simulink subsystem "cmds2forces_map"  (R2024b)
settings: Solver=VariableStepAuto  StartTime=0.0  StopTime=10.0  RelTol=1e-3
undefined symbols (not defined in the file): Parameters
libraries: eeGeneralControl x32, matrix_library x1
settings Model: Creator=thesa  LastModifiedBy=thesa
settings RTWCC: GPUComputeCapability=3.5

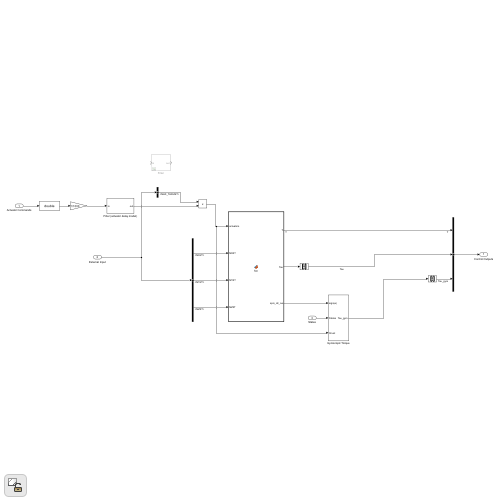
[thumbnail: Simulink's stored preview of the top-level diagram]
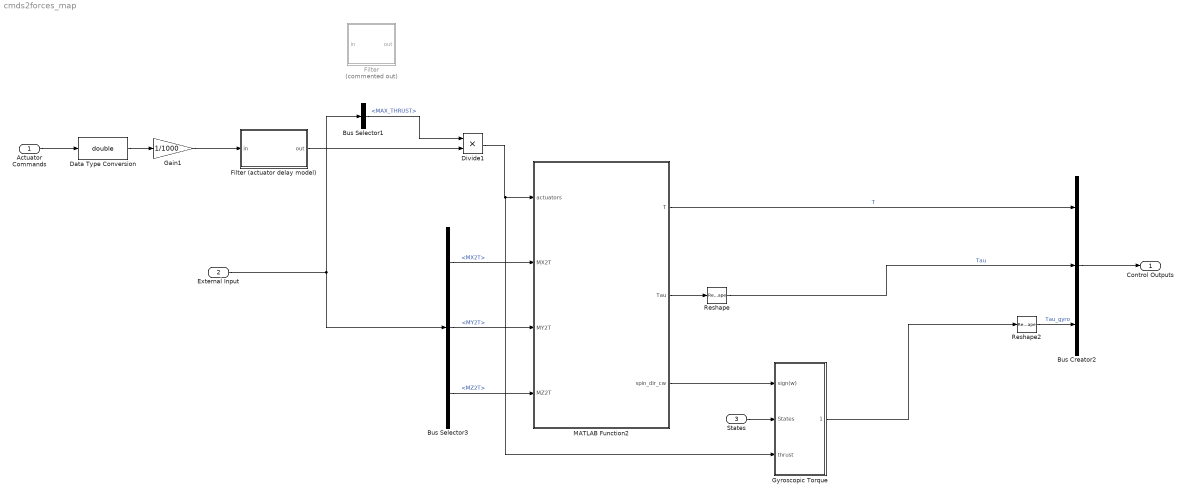
== system cmds2forces_map ==
  Actuator Commands : Inport
  External Input : Inport  Port=2
  States : Inport  Port=3
  Bus Creator2 : BusCreator  Inputs=3
  Bus Selector1 : BusSelector  OutputSignals=Vehicle Parameters.MAX_THRUST
  Bus Selector3 : BusSelector  OutputSignals=Vehicle Parameters.MX2T,Vehicle Parameters.MY2T,Vehicle Parameters.MZ2T
  Data Type Conversion : DataTypeConversion  OutDataTypeStr=double  RndMeth=Convergent  SaturateOnIntegerOverflow=off
  Divide1 : Product  Inputs=**
  Filter : Subsystem  Commented=on
  Filter (actuator delay model) : Subsystem
  Gain1 : Gain  Gain=1/1000
  Gyroscopic Torque : Subsystem
  MATLAB Function2 : MATLAB Function  TreatAsAtomicUnit=on
  Reshape : Reshape  OutputDimensionality=Column vector (2-D)
  Reshape2 : Reshape  OutputDimensionality=Column vector (2-D)
  Control Outputs : Outport
  wires:
  Data Type Conversion/1 -> Gain1/1
  Reshape/1 -> Bus Creator2/2  "Tau"
  MATLAB Function2/1(T) -> Bus Creator2/1  "T"
  External Input/1 -> Bus Selector1/1, Bus Selector3/1
  Filter (actuator delay model)/1(out) -> Divide1/2
  Bus Creator2/1 -> Control Outputs/1
  Actuator Commands/1 -> Data Type Conversion/1
  Bus Selector3/3 -> MATLAB Function2/4(MZ2T)  "<MZ2T>"
  MATLAB Function2/2(Tau) -> Reshape/1
  Divide1/1 -> MATLAB Function2/1(actuators), Gyroscopic Torque/3(thrust)
  Gain1/1 -> Filter (actuator delay model)/1(in)
  Bus Selector3/2 -> MATLAB Function2/3(MY2T)  "<MY2T>"
  Bus Selector1/1 -> Divide1/1  "<MAX_THRUST>"
  Bus Selector3/1 -> MATLAB Function2/2(MX2T)  "<MX2T>"
  Reshape2/1 -> Bus Creator2/3  "Tau_gyro"
  MATLAB Function2/3(spin_dir_cw) -> Gyroscopic Torque/1(sign(w))
  States/1 -> Gyroscopic Torque/2(States)
  Gyroscopic Torque/1(Tau_gyro) -> Reshape2/1

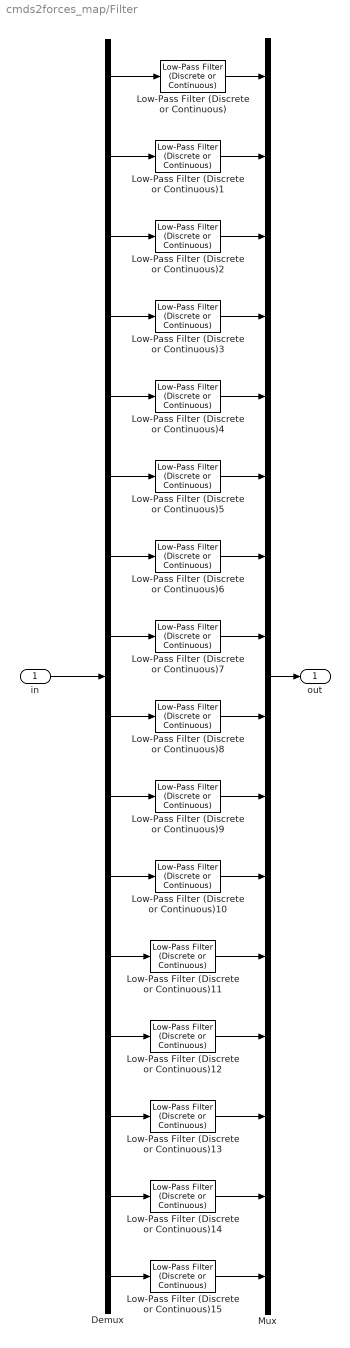
== system cmds2forces_map/Filter ==
  in : Inport
  Demux : Demux  Outputs=16
  Low-Pass Filter (Discrete or Continuous){,1..15} (16 alike) : eeGeneralControl/Low-Pass Filter (Discrete or Continuous)  K=1  T=Parameters.Vehicle.motor_time_constant_s  B=inf  A=-inf  init_option=Inherited from block input  x0=0  Ts=-1
  Mux : Mux  Inputs=16
  out : Outport
  wires:
  Low-Pass Filter (Discrete or Continuous)2/1 -> Mux/3
  Low-Pass Filter (Discrete or Continuous)/1 -> Mux/1
  Demux/3 -> Low-Pass Filter (Discrete or Continuous)2/1
  in/1 -> Demux/1
  Mux/1 -> out/1
  Low-Pass Filter (Discrete or Continuous)1/1 -> Mux/2
  Demux/1 -> Low-Pass Filter (Discrete or Continuous)/1
  Demux/2 -> Low-Pass Filter (Discrete or Continuous)1/1
  Demux/4 -> Low-Pass Filter (Discrete or Continuous)3/1
  Low-Pass Filter (Discrete or Continuous)3/1 -> Mux/4
  Demux/5 -> Low-Pass Filter (Discrete or Continuous)4/1
  Low-Pass Filter (Discrete or Continuous)4/1 -> Mux/5
  Demux/6 -> Low-Pass Filter (Discrete or Continuous)5/1
  Low-Pass Filter (Discrete or Continuous)5/1 -> Mux/6
  Low-Pass Filter (Discrete or Continuous)6/1 -> Mux/7
  Demux/7 -> Low-Pass Filter (Discrete or Continuous)6/1
  Demux/8 -> Low-Pass Filter (Discrete or Continuous)7/1
  Low-Pass Filter (Discrete or Continuous)7/1 -> Mux/8
  Demux/9 -> Low-Pass Filter (Discrete or Continuous)8/1
  Low-Pass Filter (Discrete or Continuous)8/1 -> Mux/9
  Demux/10 -> Low-Pass Filter (Discrete or Continuous)9/1
  Low-Pass Filter (Discrete or Continuous)9/1 -> Mux/10
  Demux/11 -> Low-Pass Filter (Discrete or Continuous)10/1
  Low-Pass Filter (Discrete or Continuous)10/1 -> Mux/11
  Demux/12 -> Low-Pass Filter (Discrete or Continuous)11/1
  Low-Pass Filter (Discrete or Continuous)11/1 -> Mux/12
  Demux/13 -> Low-Pass Filter (Discrete or Continuous)12/1
  Low-Pass Filter (Discrete or Continuous)12/1 -> Mux/13
  Demux/14 -> Low-Pass Filter (Discrete or Continuous)13/1
  Low-Pass Filter (Discrete or Continuous)13/1 -> Mux/14
  Demux/15 -> Low-Pass Filter (Discrete or Continuous)14/1
  Low-Pass Filter (Discrete or Continuous)14/1 -> Mux/15
  Demux/16 -> Low-Pass Filter (Discrete or Continuous)15/1
  Low-Pass Filter (Discrete or Continuous)15/1 -> Mux/16

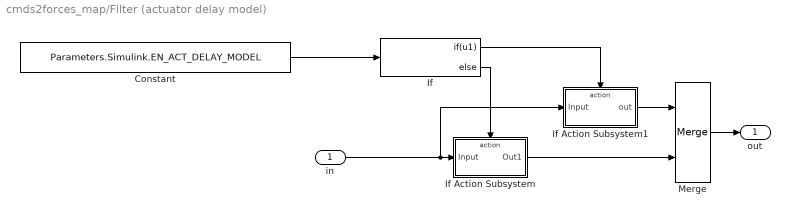
== system cmds2forces_map/Filter (actuator delay model) ==
  in : Inport
  Constant : Constant  Value=Parameters.Simulink.EN_ACT_DELAY_MODEL
  If : If  IfExpression=u1
  If Action Subsystem : Subsystem  TreatAsAtomicUnit=on
  If Action Subsystem1 : Subsystem  TreatAsAtomicUnit=on
  Merge : Merge
  out : Outport
  wires:
  If Action Subsystem/1(Out1) -> Merge/2
  in/1 -> If Action Subsystem/1(Input), If Action Subsystem1/1(Input)
  If Action Subsystem1/1(out) -> Merge/1
  If/2 -> If Action Subsystem/Action
  Constant/1 -> If/1
  If/1 -> If Action Subsystem1/Action
  Merge/1 -> out/1

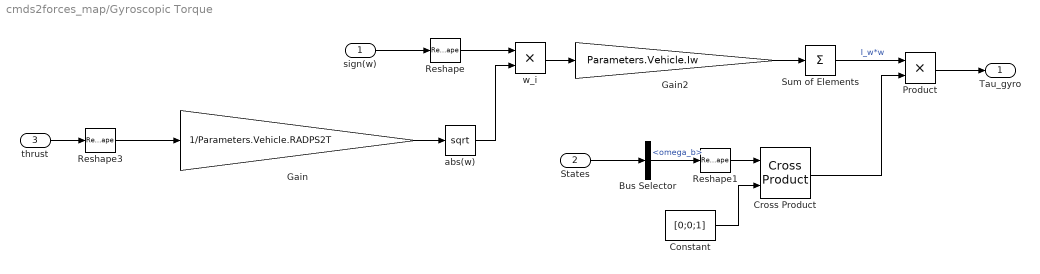
== system cmds2forces_map/Gyroscopic Torque ==
  sign(w) : Inport
  States : Inport  Port=2
  thrust : Inport  Port=3
  Bus Selector : BusSelector  OutputSignals=omega_b
  Constant : Constant  Value=[0;0;1]
  Cross Product : matrix_library/Cross Product
  Gain : Gain  Gain=1/Parameters.Vehicle.RADPS2T
  Gain2 : Gain  Gain=Parameters.Vehicle.Iw
  Product : Product
  Reshape : Reshape
  Reshape1 : Reshape  OutputDimensionality=Column vector (2-D)
  Reshape3 : Reshape
  Sum of Elements : Sum  Inputs=+
  abs(w) : Sqrt  OutputSignalType=real
  w_i : Product  Inputs=**
  Tau_gyro : Outport
  wires:
  sign(w)/1 -> Reshape/1
  Reshape3/1 -> Gain/1
  Gain2/1 -> Sum of Elements/1
  Gain/1 -> abs(w)/1
  Sum of Elements/1 -> Product/1  "I_w*w"
  Cross Product/1 -> Product/2
  Product/1 -> Tau_gyro/1
  w_i/1 -> Gain2/1
  Constant/1 -> Cross Product/2
  abs(w)/1 -> w_i/2
  Reshape/1 -> w_i/1
  Bus Selector/1 -> Reshape1/1  "<omega_b>"
  thrust/1 -> Reshape3/1
  Reshape1/1 -> Cross Product/1
  States/1 -> Bus Selector/1

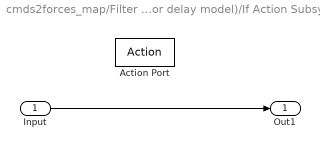
== system cmds2forces_map/Filter (actuator delay model)/If Action Subsystem ==
  Input : Inport
  Action Port : ActionPort  InitializeStates=reset
  Out1 : Outport
  wires:
  Input/1 -> Out1/1

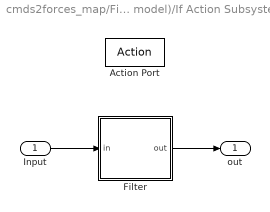
== system cmds2forces_map/Filter (actuator delay model)/If Action Subsystem1 ==
  Input : Inport
  Action Port : ActionPort  InitializeStates=reset
  Filter : Subsystem
  out : Outport
  wires:
  Filter/1(out) -> out/1
  Input/1 -> Filter/1(in)

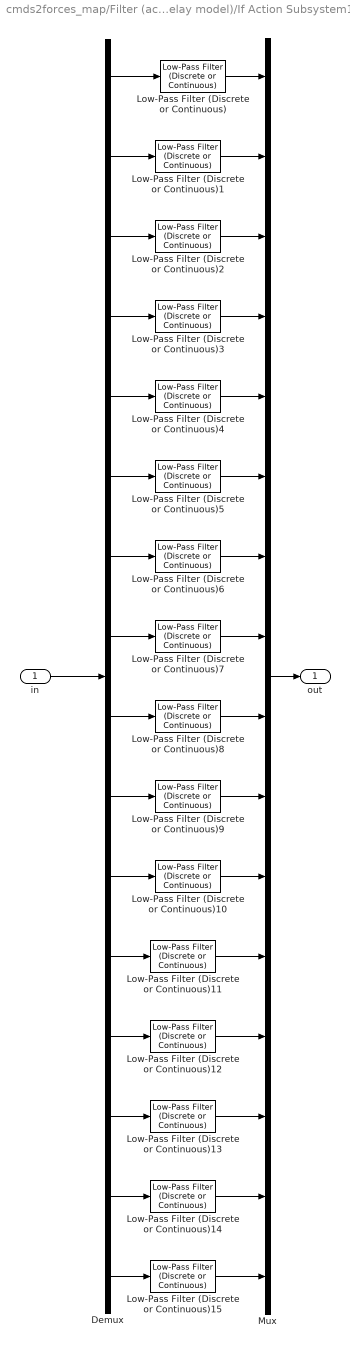
== system cmds2forces_map/Filter (actuator delay model)/If Action Subsystem1/Filter ==
  in : Inport
  Demux : Demux  Outputs=16
  Low-Pass Filter (Discrete or Continuous){,1..15} (16 alike) : eeGeneralControl/Low-Pass Filter (Discrete or Continuous)  K=1  T=Parameters.Vehicle.motor_time_constant_s  B=inf  A=-inf  init_option=Inherited from block input  x0=0  Ts=-1
  Mux : Mux  Inputs=16
  out : Outport
  wires:
  Low-Pass Filter (Discrete or Continuous)2/1 -> Mux/3
  Low-Pass Filter (Discrete or Continuous)/1 -> Mux/1
  Demux/3 -> Low-Pass Filter (Discrete or Continuous)2/1
  in/1 -> Demux/1
  Mux/1 -> out/1
  Low-Pass Filter (Discrete or Continuous)1/1 -> Mux/2
  Demux/1 -> Low-Pass Filter (Discrete or Continuous)/1
  Demux/2 -> Low-Pass Filter (Discrete or Continuous)1/1
  Demux/4 -> Low-Pass Filter (Discrete or Continuous)3/1
  Low-Pass Filter (Discrete or Continuous)3/1 -> Mux/4
  Demux/5 -> Low-Pass Filter (Discrete or Continuous)4/1
  Low-Pass Filter (Discrete or Continuous)4/1 -> Mux/5
  Demux/6 -> Low-Pass Filter (Discrete or Continuous)5/1
  Low-Pass Filter (Discrete or Continuous)5/1 -> Mux/6
  Low-Pass Filter (Discrete or Continuous)6/1 -> Mux/7
  Demux/7 -> Low-Pass Filter (Discrete or Continuous)6/1
  Demux/8 -> Low-Pass Filter (Discrete or Continuous)7/1
  Low-Pass Filter (Discrete or Continuous)7/1 -> Mux/8
  Demux/9 -> Low-Pass Filter (Discrete or Continuous)8/1
  Low-Pass Filter (Discrete or Continuous)8/1 -> Mux/9
  Demux/10 -> Low-Pass Filter (Discrete or Continuous)9/1
  Low-Pass Filter (Discrete or Continuous)9/1 -> Mux/10
  Demux/11 -> Low-Pass Filter (Discrete or Continuous)10/1
  Low-Pass Filter (Discrete or Continuous)10/1 -> Mux/11
  Demux/12 -> Low-Pass Filter (Discrete or Continuous)11/1
  Low-Pass Filter (Discrete or Continuous)11/1 -> Mux/12
  Demux/13 -> Low-Pass Filter (Discrete or Continuous)12/1
  Low-Pass Filter (Discrete or Continuous)12/1 -> Mux/13
  Demux/14 -> Low-Pass Filter (Discrete or Continuous)13/1
  Low-Pass Filter (Discrete or Continuous)13/1 -> Mux/14
  Demux/15 -> Low-Pass Filter (Discrete or Continuous)14/1
  Low-Pass Filter (Discrete or Continuous)14/1 -> Mux/15
  Demux/16 -> Low-Pass Filter (Discrete or Continuous)15/1
  Low-Pass Filter (Discrete or Continuous)15/1 -> Mux/16

== matlab function cmds2forces_map/MATLAB Function2 ==
  data: actuators input; T output; MX2T input; MY2T input; MZ2T input; Tau output; spin_dir_cw output
function [T, Tau, spin_dir_cw]  = fcn(actuators, ...
    MX2T, MY2T, MZ2T)

THRUST_IND  = 1;
ROLL_IND    = 2;
PITCH_IND   = 3;
YAW_IND     = 4;

%{
Quadrotor X:
3-cw    1-ccw
    X
    /\
    ||
    -Z ====>Y

2-ccw   4-cw
%}
motor_mixing_ = ...
    [...
    -1, -MX2T, MY2T, MZ2T
    -1, MX2T, -MY2T, MZ2T
    -1, MX2T, MY2T, -MZ2T
    -1, -MX2T, -MY2T, -MZ2T];
[nMotors, nDOFs] = size(motor_mixing_);

spin_dir_cw = zeros(1,16);
[n_,~] = size(motor_mixing_);

spin_dir_cw(1:n_) = sign(-motor_mixing_(1:n_,4));

[T, Tau] = mix_motors_(actuators, motor_mixing_);


    function [T, Tau] = mix_motors_(Control_Output, motor_mixing)
        Tau = zeros(3,1);
        T = 0;

        for i_actuator_ = 1:nMotors
            T = T + 1/motor_mixing(i_actuator_, THRUST_IND)*Control_Output(i_actuator_);
            Tau(1) = Tau(1) + 1/motor_mixing(i_actuator_, ROLL_IND)*Control_Output(i_actuator_);
            Tau(2) = Tau(2) + 1/motor_mixing(i_actuator_, PITCH_IND)*Control_Output(i_actuator_);
            Tau(3) = Tau(3) + 1/motor_mixing(i_actuator_, YAW_IND)*Control_Output(i_actuator_);
        end
    end
end
